simulink model "task_3_sim"  (R2022b)
settings: Solver=VariableStepAuto  StartTime=0.0  StopTime=10.0  RelTol=1e-3
model workspace (MAT data in the model file):
  C0 = [1  0  0  0  0  0; 0  1  0  0  0  0; 0  0  1  0  0  0; 0  0  0  1  0  0; 0  0  0  0  1  0; 0  0  0  0  0  1]
  D0 = [0  0; 0  0; 0  0; 0  0; 0  0; 0  0]
values from neighbouring files (symbols this model uses):
  C = [C, chooseCol]    [turnToControllableCanonicalForm.m]
undefined symbols (not defined in the file or in its folder): A, B, L3_1, x0
settings Model: Creator=小灰  LastModifiedBy=小灰

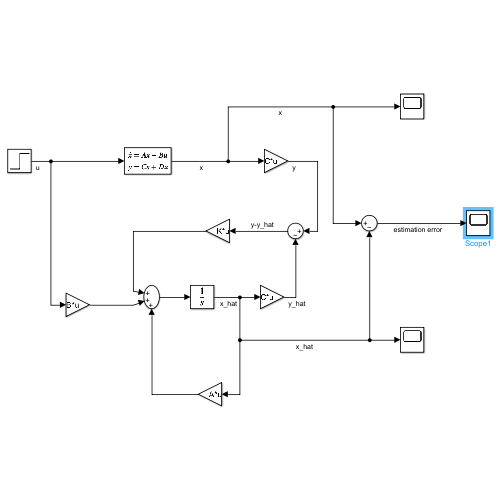
[thumbnail: Simulink's stored preview of the top-level diagram]
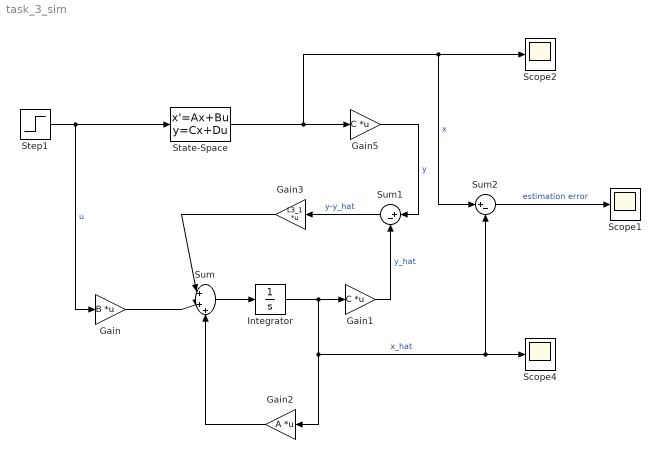
== system task_3_sim ==
  Gain : Gain  Gain=B  Multiplication=Matrix(K*u)
  Gain1 : Gain  Gain=C  Multiplication=Matrix(K*u)
  Gain2 : Gain  Gain=A  Multiplication=Matrix(K*u)
  Gain3 : Gain  Gain=L3_1  Multiplication=Matrix(K*u)
  Gain5 : Gain  Gain=C  Multiplication=Matrix(K*u)
  Integrator : Integrator
  Scope1 : Scope
  Scope2 : Scope
  Scope4 : Scope
  State-Space : StateSpace  A=A  B=B  C=C0  D=D0  InitialCondition=x0  ParameterTunability=Unconstrained
  Step1 : Step  Before=[0, 0]  After=[0, 0]  SampleTime=0
  Sum : Sum  Inputs=|+++
  Sum1 : Sum  Inputs=|+-
  Sum2 : Sum  Inputs=|+-
  wires:
  Gain5/1 -> Sum1/1  "y"
  State-Space/1 -> Gain5/1, Sum2/1, Scope2/1  "x"
  Integrator/1 -> Gain1/1, Gain2/1, Sum2/2, Scope4/1  "x_hat"
  Sum/1 -> Integrator/1
  Gain2/1 -> Sum/3
  Gain/1 -> Sum/2
  Gain1/1 -> Sum1/2  "y_hat"
  Sum1/1 -> Gain3/1  "y-y_hat"
  Gain3/1 -> Sum/1
  Step1/1 -> Gain/1, State-Space/1  "u"
  Sum2/1 -> Scope1/1  "estimation error"
